simulink model "MEEN432_Project2_Wk3"  (R2023b)
settings: Solver=VariableStepAuto  StartTime=0.0  StopTime=305  RelTol=1e-3
values from neighbouring files (symbols this model uses):
  alpha_max = 8 * pi/180    (= 0.13962634016)    [MEEN432_Project2_init.m]
  C_alphaf = 40000    [MEEN432_Project2_init.m]
  C_alphar = 40000    [MEEN432_Project2_init.m]
  Fyf_max = 40000*1/180*pi    (= 698.131700798)    [MEEN432_Project2_init.m]
  Fyr_max = 40000*1/180*pi    (= 698.131700798)    [MEEN432_Project2_init.m]
  inertia = 1600    [MEEN432_Project2_init.m]
  lf = 1.5    [MEEN432_Project2_init.m]
  lookahead_dist = 10    [MEEN432_Project2_init.m]
  lr = 1.0    (= 1)    [MEEN432_Project2_init.m]
  mass = 1000    [MEEN432_Project2_init.m]
  omega0 = 0    [MEEN432_Project2_init.m]
  psi0 = 0    [MEEN432_Project2_init.m]
  vd = 10    [MEEN432_Project2_init.m]
  vy0 = 0    [MEEN432_Project2_init.m]
  X0 = 0    [MEEN432_Project2_init.m]
  Y0 = 0    [MEEN432_Project2_init.m]
undefined symbols (not defined in the file or in its folder): x_track, y_track
settings Model: Creator=flare  LastModifiedBy=flare
settings DataIOCC: ReturnWorkspaceOutputsName=carsim

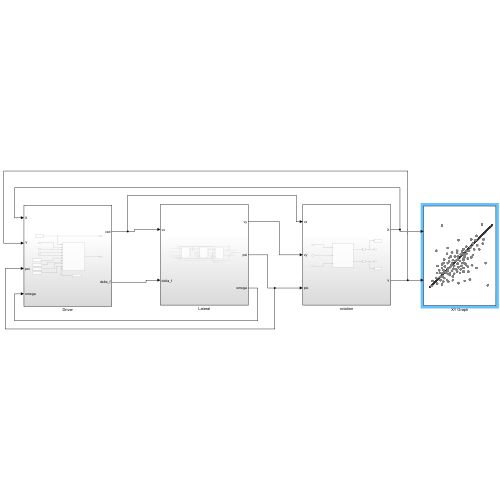
[thumbnail: Simulink's stored preview of the top-level diagram]
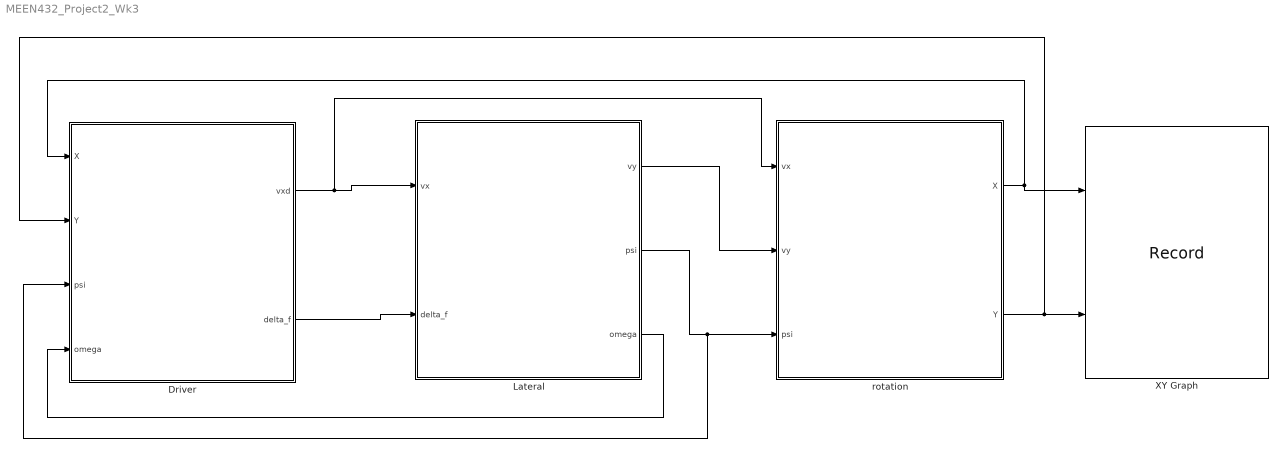
== system MEEN432_Project2_Wk3 ==
  Driver : Subsystem
  Lateral : Subsystem
  XY Graph : Record  FileSettingsInternal="{\"entries\":[{\"content\":{\"excelSettings\":{\"content\":{},\"type\":\"Streamout.ExcelSettings\"}},\"type\":\"Streamout.FileSettingStorage\",\"uuid\":\"\"}],\"packageUris\":[\"http:\\/\\/schema.mathworks.com\\/mf0\\/streamout_blocks\\/R2020a\"],\"version\":\"1.0\"}"  Layout=[1 1]  SignalsInternal="{\"entries\":[{\"content\":{\"signals\":[{\"content\":{\"blockPath\":[],\"dimensions\":[1],\"domain\":\"\",\"lineColor\":\"#a2142f\",\"plots\":[1],\"port\":1,\"sid\":[\"\"],\"signalID\":528,\"signalName\":\"rotation:1\"},\"type\":\"RecordBlkView.Signal\",\"uuid\":\"\"},{\"content\":{\"blockPath\":[],\"dimensions\":[1],\"domain\":\"\",\"lineColor\":\"#139fff\",\"plots\":[1],\"port\":2,\"sid\":[\"\"],\"signalID\":532,\"signalName\":\"rotation:2\"},\"type\":\"RecordBlkView.Signal\",\"uuid\":\"\"}]},\"type\":\"RecordBlkView.InputSignals\",\"uuid\":\"\"}],\"packageUris\":[\"http:\\/\\/schema.mathworks.com\\/mf0\\/streamout_blocks\\/R2020a\"],\"version\":\"1.0\"}"  VisualizationBindings="{\"xyplotplugin\":{\"info\":[{\"series\":[{\"bindingParametersList\":[{\"parameter\":\"X-Axis\",\"signalID\":528,\"signalName\":\"rotation:1\"},{\"parameter\":\"Y-Axis\",\"signalID\":532,\"signalName\":\"rotation:2\"}],\"seriesID\":60233}],\"subplotID\":1}]}}"  CompatibilityTag=XY
  rotation : Subsystem
  wires:
  Driver/1(vxd) -> rotation/1(vx), Lateral/1(vx)
  Driver/2(delta_f) -> Lateral/2(delta_f)
  Lateral/2(psi) -> Driver/3(psi), rotation/3(psi)
  Lateral/1(vy) -> rotation/2(vy)
  Lateral/3(omega) -> Driver/4(omega)
  rotation/1(X) -> Driver/1(X), XY Graph/1
  rotation/2(Y) -> Driver/2(Y), XY Graph/2

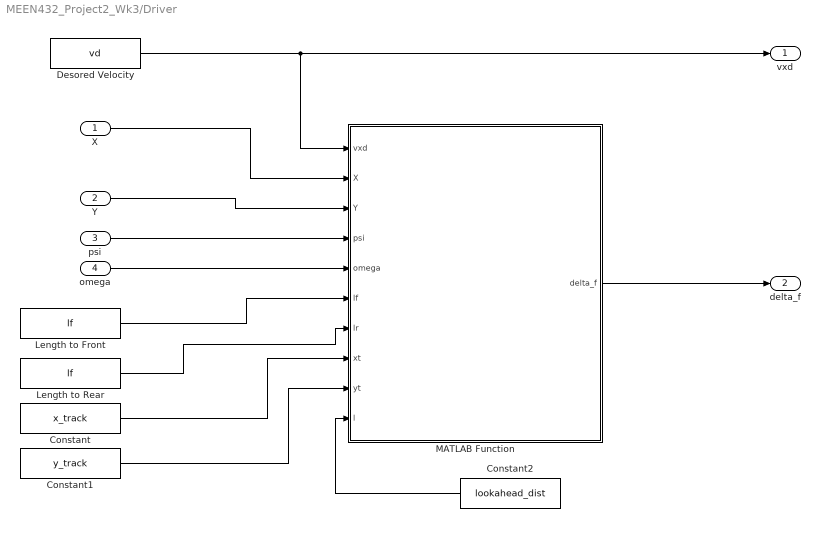
== system MEEN432_Project2_Wk3/Driver ==
  X : Inport
  Y : Inport  Port=2
  psi : Inport  Port=3
  omega : Inport  Port=4
  Constant : Constant  Value=x_track  VectorParams1D=off
  Constant1 : Constant  Value=y_track  VectorParams1D=off
  Constant2 : Constant  Value=lookahead_dist
  Desored Velocity : Constant  Value=vd
  Length to Front : Constant  Value=lf
  Length to Rear : Constant  Value=lf
  MATLAB Function : MATLAB Function  TreatAsAtomicUnit=on
  vxd : Outport
  delta_f : Outport  Port=2
  wires:
  omega/1 -> MATLAB Function/5(omega)
  psi/1 -> MATLAB Function/4(psi)
  Y/1 -> MATLAB Function/3(Y)
  X/1 -> MATLAB Function/2(X)
  Length to Front/1 -> MATLAB Function/6(lf)
  Constant/1 -> MATLAB Function/8(xt)
  Constant1/1 -> MATLAB Function/9(yt)
  Desored Velocity/1 -> vxd/1, MATLAB Function/1(vxd)
  MATLAB Function/1(delta_f) -> delta_f/1
  Constant2/1 -> MATLAB Function/10(l)
  Length to Rear/1 -> MATLAB Function/7(lr)

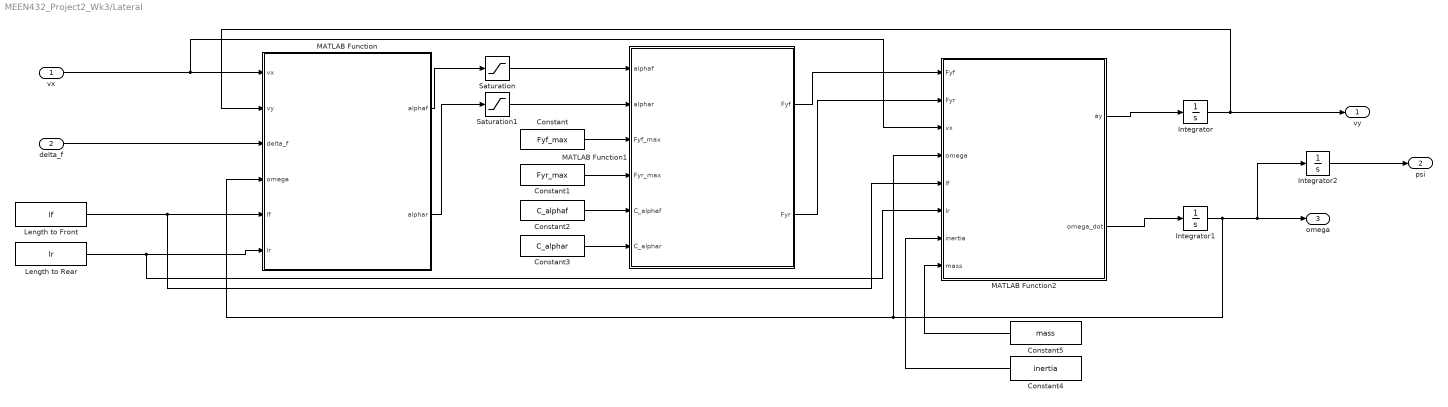
== system MEEN432_Project2_Wk3/Lateral ==
  vx : Inport
  delta_f : Inport  Port=2
  Constant : Constant  Value=Fyf_max
  Constant1 : Constant  Value=Fyr_max
  Constant2 : Constant  Value=C_alphaf
  Constant3 : Constant  Value=C_alphar
  Constant4 : Constant  Value=inertia
  Constant5 : Constant  Value=mass
  Integrator : Integrator  InitialCondition=vy0
  Integrator1 : Integrator  InitialCondition=omega0
  Integrator2 : Integrator  InitialCondition=psi0
  Length to Front : Constant  Value=lf
  Length to Rear : Constant  Value=lr
  MATLAB Function : MATLAB Function  TreatAsAtomicUnit=on
  MATLAB Function1 : MATLAB Function  TreatAsAtomicUnit=on
  MATLAB Function2 : MATLAB Function  TreatAsAtomicUnit=on
  Saturation : Saturate  UpperLimit=alpha_max  LowerLimit=-alpha_max
  Saturation1 : Saturate  UpperLimit=alpha_max  LowerLimit=-alpha_max
  vy : Outport
  psi : Outport  Port=2
  omega : Outport  Port=3
  wires:
  vx/1 -> MATLAB Function2/3(vx), MATLAB Function/1(vx)
  delta_f/1 -> MATLAB Function/3(delta_f)
  MATLAB Function/1(alphaf) -> Saturation/1
  MATLAB Function/2(alphar) -> Saturation1/1
  Saturation/1 -> MATLAB Function1/1(alphaf)
  Saturation1/1 -> MATLAB Function1/2(alphar)
  MATLAB Function1/1(Fyf) -> MATLAB Function2/1(Fyf)
  MATLAB Function1/2(Fyr) -> MATLAB Function2/2(Fyr)
  MATLAB Function2/1(ay) -> Integrator/1
  MATLAB Function2/2(omega_dot) -> Integrator1/1
  Integrator1/1 -> MATLAB Function/4(omega), MATLAB Function2/4(omega), omega/1, Integrator2/1
  Integrator/1 -> MATLAB Function/2(vy), vy/1
  Integrator2/1 -> psi/1
  Length to Front/1 -> MATLAB Function2/5(lf), MATLAB Function/5(lf)
  Length to Rear/1 -> MATLAB Function2/6(lr), MATLAB Function/6(lr)
  Constant/1 -> MATLAB Function1/3(Fyf_max)
  Constant1/1 -> MATLAB Function1/4(Fyr_max)
  Constant2/1 -> MATLAB Function1/5(C_alphaf)
  Constant3/1 -> MATLAB Function1/6(C_alphar)
  Constant4/1 -> MATLAB Function2/7(inertia)
  Constant5/1 -> MATLAB Function2/8(mass)

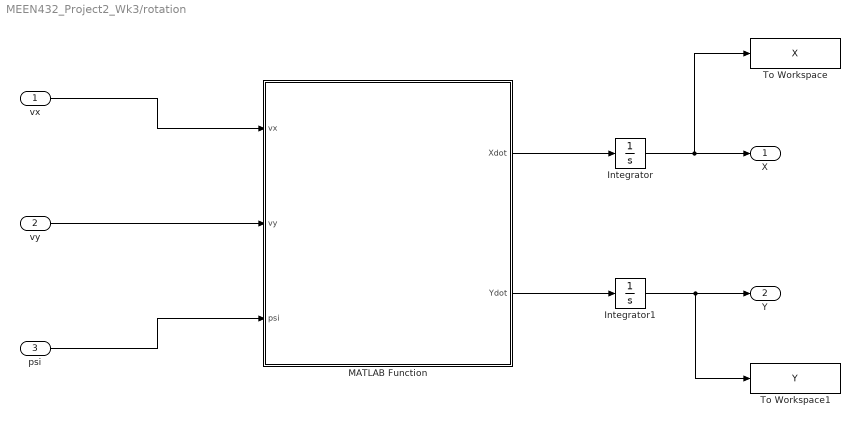
== system MEEN432_Project2_Wk3/rotation ==
  vx : Inport
  vy : Inport  Port=2
  psi : Inport  Port=3
  Integrator : Integrator  InitialCondition=X0
  Integrator1 : Integrator  InitialCondition=Y0
  MATLAB Function : MATLAB Function  TreatAsAtomicUnit=on
  To Workspace : ToWorkspace  VariableName=X  SaveFormat=Timeseries  SampleTime=-1
  To Workspace1 : ToWorkspace  VariableName=Y  SaveFormat=Timeseries  SampleTime=-1
  X : Outport
  Y : Outport  Port=2
  wires:
  vx/1 -> MATLAB Function/1(vx)
  vy/1 -> MATLAB Function/2(vy)
  psi/1 -> MATLAB Function/3(psi)
  MATLAB Function/1(Xdot) -> Integrator/1
  MATLAB Function/2(Ydot) -> Integrator1/1
  Integrator/1 -> To Workspace/1, X/1
  Integrator1/1 -> To Workspace1/1, Y/1

== matlab function MEEN432_Project2_Wk3/Lateral/MATLAB Function ==
  data: vx input; vy input; alphaf output; delta_f input; omega input; alphar output; vx_max parameter; lf input; lr input
function [alphaf, alphar] = fcn(vx, vy, delta_f, omega, vx_max, lf, lr)

%make sure velocity isn't too high
if abs(vx) > vx_max
    alphaf = delta_f - (vy + omega *lf) / vx;
    alphar = -(vy - omega *lr) / vx;
else
    alphaf = 0;
    alphar = 0;
end

== matlab function MEEN432_Project2_Wk3/Driver/MATLAB Function ==
  data: vxd input; X input; delta_f output; Y input; psi input; omega input; lf input; lr input; xt input; yt input; l input
function delta_f = fcn(vxd, X, Y, psi, omega, lf, lr, xt, yt, l)

%initializes this function
car_loc = [X, Y];
track = [xt; yt];
dist = [];
look_ahead = l;
base = lf + lr;

%distance to all points on track
for i = 1:length(track)
    dist(end+1) = ((track(1,i)-car_loc(1))^2 + (track(2,i) - car_loc(2))^2)^(1/2);
end

%finds closest point and adds the set look ahead distance
[~, closest] = min(dist);
indx = closest + look_ahead;

if indx > length(track)
    indx = length(track);
end

target = track(:,indx);

%calculations
alpha = atan2(target(2)-car_loc(2), target(1)-car_loc(1)) - psi;
psi_dot = 2*vxd*sin(alpha)/base;
delta_f = psi_dot - omega;

== matlab function MEEN432_Project2_Wk3/Lateral/MATLAB Function1 ==
  data: alphaf input; Fyf output; alphar input; Fyf_max input; Fyr output; Fyr_max input; C_alphaf input; C_alphar input
function [Fyf, Fyr] = fcn(alphaf, alphar, Fyf_max, Fyr_max, C_alphaf, C_alphar)

Fyf = C_alphaf * alphaf;
Fyr = C_alphar * alphar;

if Fyf > Fyf_max
    Fyf = Fyf_max;
end

if Fyr > Fyr_max
    Fyr = Fyr_max;
end

== matlab function MEEN432_Project2_Wk3/Lateral/MATLAB Function2 ==
  data: Fyf input; ay output; Fyr input; vx input; omega input; omega_dot output; lf input; lr input; inertia input; mass input
function [ay, omega_dot] = fcn(Fyf, Fyr, vx, omega, lf, lr, inertia, mass)

ay = (Fyf +Fyr)/mass - omega*vx;

M = Fyf*lf - Fyr*lr;
omega_dot = M/inertia;

== matlab function MEEN432_Project2_Wk3/rotation/MATLAB Function ==
  data: vx input; Xdot output; vy input; psi input; Ydot output
function [Xdot, Ydot] = fcn(vx, vy, psi)

%velocity matrix
v = [vx; vy];
%rotation matrix
rot = [cos(psi), -sin(psi); sin(psi), cos(psi)];

temp = rot * v;

%rotated velocity matrix
Xdot = temp(1);
Ydot = temp(2);
